simulink model "absbrake"  (Simulink 6.0)
settings: Solver=ode45  SolverMode=SingleTasking  StartTime=0.0  StopTime=5  MaxStep=.01  RelTol=1e-3  AbsTol=1e-6
PreLoadFcn:
  | absdata
values from neighbouring files (symbols this model uses):
  g = 9.8    [DATA.m]
  I = 5    [DATA.m]
  Kf = 1    [DATA.m]
  m = 300    [DATA.m]
  mu = [0 .4 .8 .97 1.0 .98 .96 .94 .92 .9 .88 .855 .83 .81 .79 .77 .75 .73 .72 .71 .7]    [DATA.m]
  PBmax = 1500    [DATA.m]
  Rr = 0.35    [DATA.m]
  slip = (0:.05:1.0)    [DATA.m]
  TB = 0.01    [DATA.m]
  v0 = 25    [DATA.m]
libraries: fuzblock x1
settings Model: Creator=ctrapeni  LastModifiedBy=xiangxiang  ExtModeTrigMode=oneshot  ExtModeArmWhenConnect=off
settings DataIOCC: LimitDataPoints=off  SaveOutput=off  TimeSaveName=time
settings OptimizationCC: BlockReduction=off  BooleanDataType=off  InlineInvariantSignals=off
settings DebuggingCC: SolverPrmCheckMsg=none  IntegerOverflowMsg=none
settings HardwareCC: TargetUnknown=on

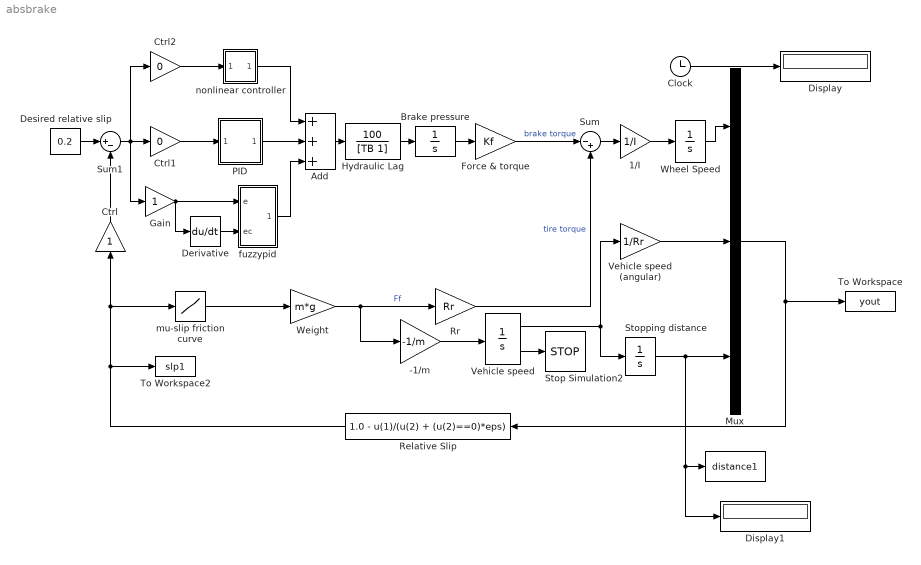
== system absbrake ==
  " " : ToWorkspace  VariableName=distance1  SampleTime=-1  SaveFormat=Array
  -1/m : Gain  Gain=-1/m  SaturateOnIntegerOverflow=on
  1/I : Gain  Gain=1/I  SaturateOnIntegerOverflow=on
  Add : Sum  Inputs=+++  OutScaling=2^-10
  Brake pressure : Integrator  LimitOutput=on  UpperSaturationLimit=PBmax  LowerSaturationLimit=0
  Clock : Clock
      settings: Decimation=10
  Ctrl : Gain  Orientation=up  SaturateOnIntegerOverflow=on
  Ctrl1 : Gain  Gain=0  SaturateOnIntegerOverflow=on
  Ctrl2 : Gain  Gain=0  SaturateOnIntegerOverflow=on
  Derivative : Derivative
  Desired relative slip : Constant  Value=0.2
  Display : Display
  Display1 : Display
  Force & torque : Gain  Gain=Kf  SaturateOnIntegerOverflow=on
  Gain : Gain
  "Hydraulic Lag " : TransferFcn  Numerator=[100]  Denominator=[TB 1]
  Mux : Mux  Inputs=3
  PID : Subsystem
  Relative Slip : Fcn  Orientation=left  Expr=1.0 - u(1)/(u(2) + (u(2)==0)*eps)
  Rr : Gain  Gain=Rr  SaturateOnIntegerOverflow=on
  Stop Simulation2 : Stop
  Stopping distance : Integrator  UpperSaturationLimit=1000  LowerSaturationLimit=0
  Sum : Sum  Inputs=|-+  SaturateOnIntegerOverflow=on  InputSameDT=on
  Sum1 : Sum  Inputs=|+-  SaturateOnIntegerOverflow=on  InputSameDT=on
  To Workspace : ToWorkspace  VariableName=yout  SaveFormat=Array
      settings: MaxDataPoints=10000
  To Workspace2 : ToWorkspace  VariableName=slp1  SaveFormat=Array
      settings: MaxDataPoints=10000
  Vehicle speed : Integrator  InitialCondition=v0  LimitOutput=on  UpperSaturationLimit=500  LowerSaturationLimit=0.008  ShowSaturationPort=on
  Vehicle speed (angular) : Gain  Gain=1/Rr  SaturateOnIntegerOverflow=on
  Weight : Gain  Gain=m*g  SaturateOnIntegerOverflow=on
  Wheel Speed : Integrator  InitialCondition=v0/Rr  LimitOutput=on  UpperSaturationLimit=1000  LowerSaturationLimit=0
  fuzzypid : Subsystem
  mu-slip friction curve : Lookup  DialogController=Simulink.DDGSource  InputValues=slip  OutputValues=mu  SaturateOnIntegerOverflow=on
  nonlinear controller : Subsystem
      mask Type: Sign
      mask Description: y = sign(x)
      mask Help: Sign Function:\n\t\t\ty = 1 if x > 0\n\t\t\ty = 0 if x = 0\n\t\t\ty = -1 if x < 0
      mask Display: plot(-50,-50,50,50,[-50,50],[0,0],[0,0],[-50,50],[-40,0],[-30,-30],[0,40],[30,30])
  wires:
  1/I/1 -> Wheel Speed/1
  Mux/1 -> To Workspace/1, Relative Slip/1
  Sum/1 -> 1/I/1
  Vehicle speed (angular)/1 -> Mux/2
  Relative Slip/1 -> Ctrl/1, mu-slip friction curve/1, To Workspace2/1
  Rr/1 -> Sum/2  "tire torque"
  Force & torque/1 -> Sum/1  "brake torque"
  -1/m/1 -> Vehicle speed/1
  Vehicle speed/1 -> Vehicle speed (angular)/1, Stopping distance/1
  Weight/1 -> -1/m/1, Rr/1  "Ff"
  Brake pressure/1 -> Force & torque/1
  Ctrl/1 -> Sum1/2
  "Hydraulic Lag "/1 -> Brake pressure/1
  Desired relative slip/1 -> Sum1/1
  Vehicle speed/2 -> Stop Simulation2/1
  Sum1/1 -> Ctrl1/1, Ctrl2/1, Gain/1
  mu-slip friction curve/1 -> Weight/1
  Ctrl1/1 -> PID/1(In1)
  Ctrl2/1 -> nonlinear controller/1(in_1)
  PID/1(Out1) -> Add/2
  Add/1 -> "Hydraulic Lag "/1
  nonlinear controller/1(out_1) -> Add/1
  Wheel Speed/1 -> Mux/1
  fuzzypid/1(Out2) -> Add/3
  Derivative/1 -> fuzzypid/2(ec)
  Gain/1 -> Derivative/1, fuzzypid/1(e)
  Stopping distance/1 -> Mux/3, " "/1, Display1/1
  Clock/1 -> Display/1

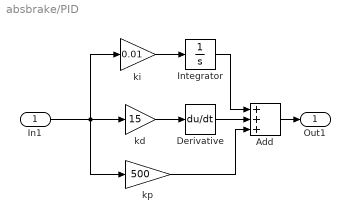
== system absbrake/PID ==
  In1 : Inport  Port=1  LatchInput=off
  Add : Sum  Inputs=+++  OutScaling=2^-10
  Derivative : Derivative
  Integrator : Integrator
  kd : Gain  Gain=15
  "ki " : Gain  Gain=0.01
  kp : Gain  Gain=500
  Out1 : Outport
  wires:
  In1/1 -> kd/1, "ki "/1, kp/1
  kd/1 -> Derivative/1
  "ki "/1 -> Integrator/1
  Add/1 -> Out1/1
  Derivative/1 -> Add/2
  Integrator/1 -> Add/1
  kp/1 -> Add/3

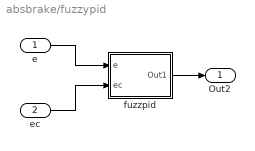
== system absbrake/fuzzypid ==
  e : Inport  Port=1  LatchInput=off
  ec : Inport  Port=2  LatchInput=off
  fuzzpid : Subsystem
  Out2 : Outport
  wires:
  fuzzpid/1(Out1) -> Out2/1
  ec/1 -> fuzzpid/2(ec)
  e/1 -> fuzzpid/1(e)

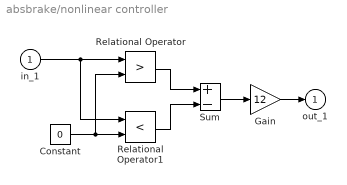
== system absbrake/nonlinear controller ==
  in_1 : Inport  Port=1  LatchInput=off
  Constant : Constant  Value=0
  Gain : Gain  Gain=12
  Relational Operator : RelationalOperator  Operator=>  InputSameDT=on
  Relational Operator1 : RelationalOperator  Operator=<  InputSameDT=on
  Sum : Sum  Inputs=+-  SaturateOnIntegerOverflow=on  InputSameDT=on
  out_1 : Outport  InitialOutput=0
  wires:
  in_1/1 -> Relational Operator/1, Relational Operator1/1
  Constant/1 -> Relational Operator1/2, Relational Operator/2
  Relational Operator1/1 -> Sum/2
  Relational Operator/1 -> Sum/1
  Gain/1 -> out_1/1
  Sum/1 -> Gain/1

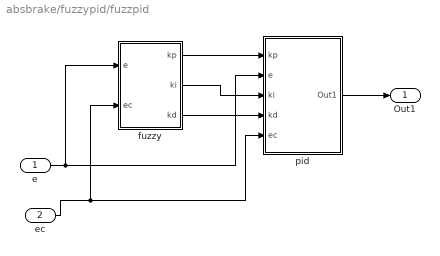
== system absbrake/fuzzypid/fuzzpid ==
  e : Inport  Port=1  LatchInput=off
  ec : Inport  Port=2  LatchInput=off
  fuzzy : Subsystem
  "pid " : Subsystem
  Out1 : Outport
  wires:
  "pid "/1(Out1) -> Out1/1
  ec/1 -> "pid "/5(ec), fuzzy/2("ec ")
  e/1 -> "pid "/2(e), fuzzy/1(e)
  fuzzy/3("kd ") -> "pid "/4("kd ")
  fuzzy/2(ki) -> "pid "/3(ki)
  fuzzy/1(kp) -> "pid "/1(kp)

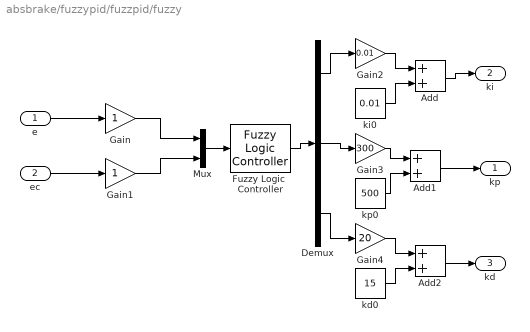
== system absbrake/fuzzypid/fuzzpid/fuzzy ==
  e : Inport  Port=1  LatchInput=off
  "ec " : Inport  Port=2  LatchInput=off
  Add : Sum  OutScaling=2^-10
  Add1 : Sum  OutScaling=2^-10
  Add2 : Sum  OutScaling=2^-10
  Demux : Demux  Outputs=3
  Fuzzy Logic  Controller : fuzblock/Fuzzy Logic  Controller  fis=FUZZYPID
  Gain : Gain
  Gain1 : Gain
  Gain2 : Gain  Gain=0.01
  Gain3 : Gain  Gain=300
  Gain4 : Gain  Gain=20
  Mux : Mux  Inputs=2
  kd0 : Constant  Value=15
  ki0 : Constant  Value=0.01
  kp0 : Constant  Value=500
  kp : Outport
  ki : Outport  Port=2
  "kd " : Outport  Port=3
  wires:
  Gain/1 -> Mux/1
  Gain1/1 -> Mux/2
  Mux/1 -> Fuzzy Logic  Controller/1
  Fuzzy Logic  Controller/1 -> Demux/1
  Demux/1 -> Gain2/1
  Demux/2 -> Gain3/1
  Demux/3 -> Gain4/1
  e/1 -> Gain/1
  "ec "/1 -> Gain1/1
  Add/1 -> ki/1
  Gain2/1 -> Add/1
  ki0/1 -> Add/2
  Gain3/1 -> Add1/1
  kp0/1 -> Add1/2
  Add1/1 -> kp/1
  Add2/1 -> "kd "/1
  Gain4/1 -> Add2/1
  kd0/1 -> Add2/2

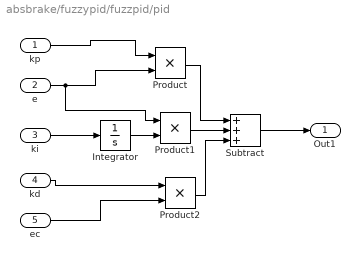
== system absbrake/fuzzypid/fuzzpid/pid  ==
  kp : Inport  Port=1  LatchInput=off
  e : Inport  Port=2  LatchInput=off
  ki : Inport  Port=3  LatchInput=off
  "kd " : Inport  Port=4  LatchInput=off
  ec : Inport  Port=5  LatchInput=off
  Integrator : Integrator
  Product : Product  RndMeth=Zero
  Product1 : Product  RndMeth=Zero
  Product2 : Product  RndMeth=Zero
  Subtract : Sum  Inputs=+++  OutScaling=2^-10
  Out1 : Outport
  wires:
  Product1/1 -> Subtract/2
  Product/1 -> Subtract/1
  Product2/1 -> Subtract/3
  Subtract/1 -> Out1/1
  e/1 -> Product/2, Product1/1
  ki/1 -> Integrator/1
  "kd "/1 -> Product2/1
  ec/1 -> Product2/2
  Integrator/1 -> Product1/2
  kp/1 -> Product/1
